simulink model "broadbandTestbed"  (R2012b)
settings: Solver=FixedStepDiscrete  StartTime=0.0  StopTime=inf  RelTol=1e-3
settings Model: BufferReuse=off  ExplicitPartitioning=on  Creator=gilja  LastModifiedBy=NPTL
settings SolverCC: EnableConcurrentExecution=on  ConcurrentTasks=on
settings OptimizationCC: InlineParams=on  InlineInvariantSignals=on  OptimizeBlockIOStorage=off  BufferReuse=off  ExpressionFolding=off  LocalBlockOutputs=off
settings HardwareCC: ProdIntDivRoundTo=Zero  ProdEndianess=LittleEndian  ProdHWDeviceType=Generic->32-bit x86 compatible
settings ModelReferenceCC: ModelReferenceMinAlgLoopOccurrences=on
settings RTWCC: SystemTargetFile=xpctarget.tlc  TemplateMakefile=xpc_default_tmf  Description=xPC Target  ProcessScript=xpctarget_make_rtw_hook
settings CodeAppCC: MaxIdLength=62
settings xpcTargetCC: TargetFcnLib=ansi_tfl_table_tmw.mat  CodeReplacementLibrary=XPC_BLAS  ParMdlRefBuildCompliant=on  ConcurrentExecutionCompliant=on  CombineSignalStateStructs=off  GRTInterface=on  xPCTaskExecutionProfile=off  xPCRL32EventNumber=5000  RL32IRQSourceModifier=5  xPCIRQSourceBoard=Parallel_Port  xPCIOIRQSlot=0x378  xPCisDownloadable=off  xPCLoadParamSetFile=off  xPCConcurrentTasks=off  xPCEnableSFAnimation=off

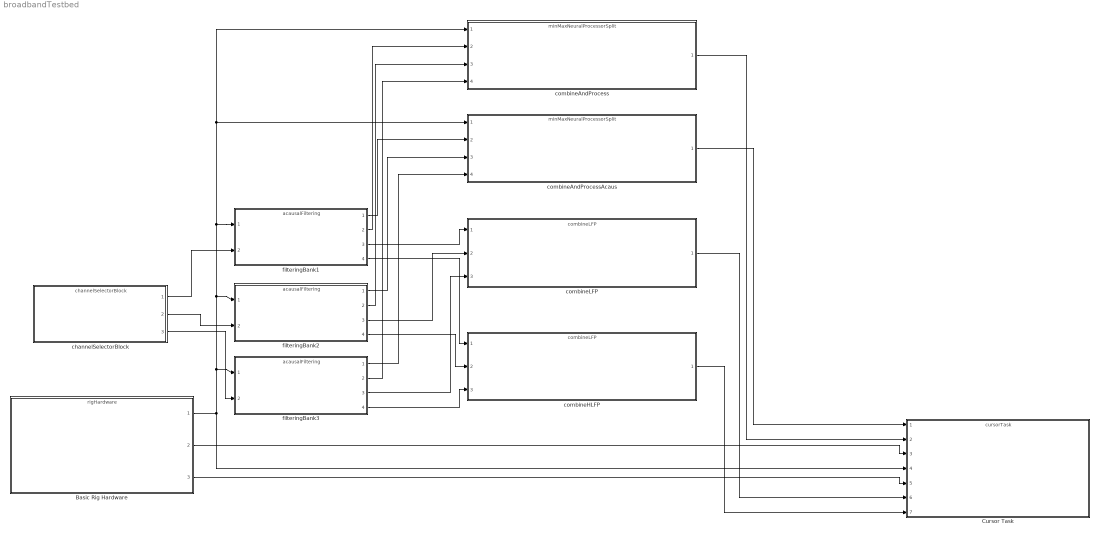
== system broadbandTestbed ==
  Basic Rig Hardware : ModelReference  ModelNameDialog=rigHardware  SimulationMode=Normal  ModelReferenceVersion=1.59  CopyOfModelName=rigHardware  DefaultDataLogging=on
  Cursor Task : ModelReference  ModelNameDialog=cursorTask  SimulationMode=Normal  ModelReferenceVersion=1.97  CopyOfModelName=cursorTask  DefaultDataLogging=on
  channelSelectorBlock : ModelReference  ModelNameDialog=channelSelectorBlock  SimulationMode=Normal  ModelReferenceVersion=1.34  CopyOfModelName=channelSelectorBlock  DefaultDataLogging=on
  combineAndProcess : ModelReference  ModelNameDialog=minMaxNeuralProcessorSplit  SimulationMode=Normal  ModelReferenceVersion=1.32  CopyOfModelName=minMaxNeuralProcessorSplit  DefaultDataLogging=on
  combineAndProcessAcaus : ModelReference  ModelNameDialog=minMaxNeuralProcessorSplit  SimulationMode=Normal  ModelReferenceVersion=1.32  CopyOfModelName=minMaxNeuralProcessorSplit  DefaultDataLogging=on
  combineHLFP : ModelReference  ModelNameDialog=combineLFP  SimulationMode=Normal  ModelReferenceVersion=1.36  CopyOfModelName=combineLFP  DefaultDataLogging=on
  combineLFP : ModelReference  ModelNameDialog=combineLFP  SimulationMode=Normal  ModelReferenceVersion=1.36  CopyOfModelName=combineLFP  DefaultDataLogging=on
  filteringBank1 : ModelReference  ModelNameDialog=acausalFiltering  SimulationMode=Normal  ModelReferenceVersion=1.45  CopyOfModelName=acausalFiltering  DefaultDataLogging=on
  filteringBank2 : ModelReference  ModelNameDialog=acausalFiltering  SimulationMode=Normal  ModelReferenceVersion=1.45  CopyOfModelName=acausalFiltering  DefaultDataLogging=on
  filteringBank3 : ModelReference  ModelNameDialog=acausalFiltering  SimulationMode=Normal  ModelReferenceVersion=1.45  CopyOfModelName=acausalFiltering  DefaultDataLogging=on
  wires:
  Basic Rig Hardware/1 -> filteringBank3/1, filteringBank2/1, combineAndProcess/1, combineAndProcessAcaus/1, filteringBank1/1, Cursor Task/4
  combineAndProcessAcaus/1 -> Cursor Task/1
  filteringBank1/1 -> combineAndProcessAcaus/2
  channelSelectorBlock/1 -> filteringBank1/2
  channelSelectorBlock/2 -> filteringBank2/2
  filteringBank2/1 -> combineAndProcessAcaus/3
  channelSelectorBlock/3 -> filteringBank3/2
  filteringBank3/1 -> combineAndProcessAcaus/4
  filteringBank1/3 -> combineLFP/1
  filteringBank2/3 -> combineLFP/2
  filteringBank3/3 -> combineLFP/3
  filteringBank1/2 -> combineAndProcess/2
  filteringBank2/2 -> combineAndProcess/3
  filteringBank3/2 -> combineAndProcess/4
  filteringBank1/4 -> combineHLFP/1
  filteringBank2/4 -> combineHLFP/2
  filteringBank3/4 -> combineHLFP/3
  combineHLFP/1 -> Cursor Task/7
  combineLFP/1 -> Cursor Task/6
  combineAndProcess/1 -> Cursor Task/2
  Basic Rig Hardware/2 -> Cursor Task/3
  Basic Rig Hardware/3 -> Cursor Task/5
